simulink model "float_vs_real"  (R2017a)
settings: Solver=FixedStepAuto  StartTime=0.0  StopTime=10.0  RelTol=1e-3
libraries: sldvlib x1
settings Model: Creator=rober  LastModifiedBy=rober
settings SolverCC: AutoInsertRateTranBlk=on

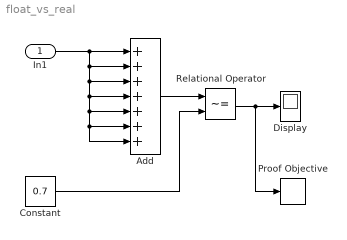
== system float_vs_real ==
  In1 : Inport  OutDataTypeStr=single
  Add : Sum  Inputs=+++++++
  Constant : Constant  Value=0.7  OutDataTypeStr=single
  Display : Display
      settings: Decimation=12
  Proof Objective : sldvlib/Objectives and Constraints/Proof Objective  enabled=on  customAVTBlockType=Proof Objective  intervals=true  dispValues=on  outEnabled=off  enableStopSim=off
      settings: AttributesFormatString=%<intervals>  SourceProductName=Simulink Design Verifier  SourceProductBaseCode=DV
  Relational Operator : RelationalOperator  Operator=~=  OutDataTypeStr=boolean  RndMeth=Simplest
  wires:
  In1/1 -> Add/3, Add/4, Add/6, Add/7, Add/5, Add/2, Add/1
  Add/1 -> Relational Operator/1
  Constant/1 -> Relational Operator/2
  Relational Operator/1 -> Proof Objective/1, Display/1
